simulink model "Ladder_Model"  (R2021b)
settings: Solver=VariableStepAuto  StartTime=0.0  StopTime=0.00005  RelTol=1e-3
model workspace (MAT data in the model file):
  f = [1 10010011.009 20020021.018 30030031.027 40040041.036 50050051.045 60060061.0541 70070071.0631 80080081.0721 90090091.0811 100100101.09 110110111.099 ... (1000 elements, 1x1000)]
  f1 = 120
  fff = Simulink.Parameter
  fff.DataType = 'auto'
  fff.Min = 0
  fff.Max = 100000
  fff.Complexity = 'real'
  fff.Dimensions = [0 0]
undefined symbols (not defined in the file or in its folder): c0, ct0, ct1, ct2, ct3, ct4, cu, cv, frequence
libraries: spsSeriesRLCBranchLib x190, spsGroundLib x49, spsControlledVoltageSourceLib x6, spsImpedanceMeasurementLib x6, spspowerguiLib x1
(part 1 of 2)
settings Model: Creator=anyon  LastModifiedBy=anyon
settings DebuggingCC: UnconnectedInputMsg=none  UnconnectedOutputMsg=none  UnconnectedLineMsg=none

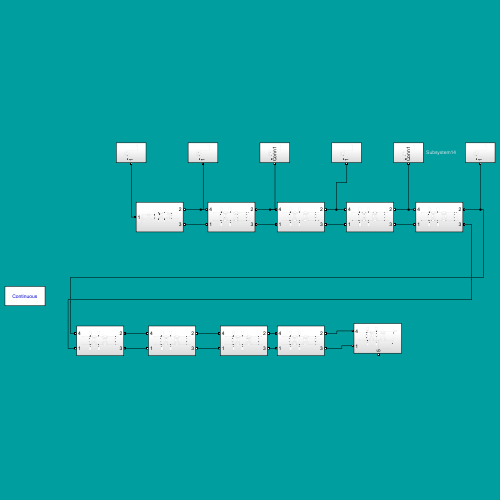
[thumbnail: Simulink's stored preview of the top-level diagram]
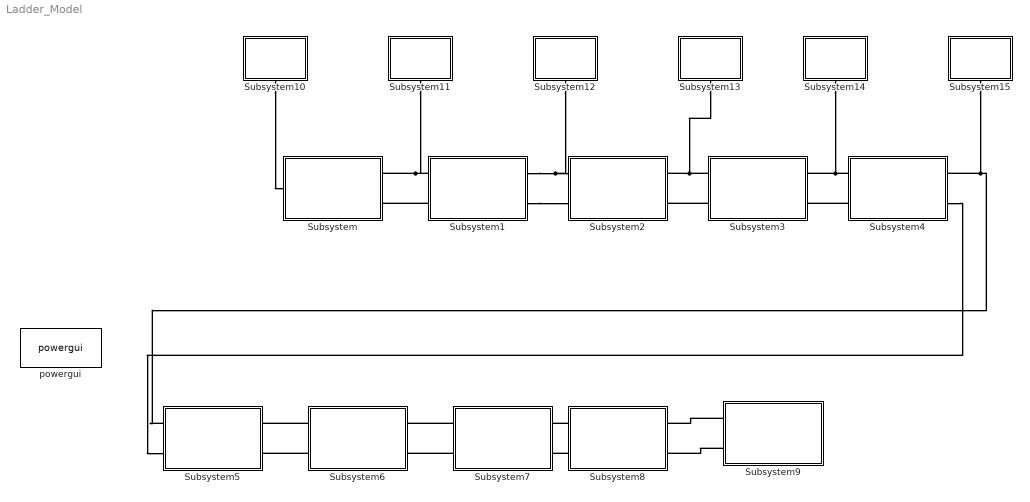
== system Ladder_Model ==
  Subsystem : Subsystem
  Subsystem1 : Subsystem
  Subsystem10 : Subsystem
  Subsystem11 : Subsystem
  Subsystem12 : Subsystem
  Subsystem13 : Subsystem
  Subsystem14 : Subsystem
  Subsystem15 : Subsystem
  Subsystem2 : Subsystem
  Subsystem3 : Subsystem
  Subsystem4 : Subsystem
  Subsystem5 : Subsystem
  Subsystem6 : Subsystem
  Subsystem7 : Subsystem
  Subsystem8 : Subsystem
  Subsystem9 : Subsystem
      settings: PortSchema="{\"entries\":[{\"content\":{\"sides\":[{\"content\":{\"connectorIds\":[\"LConn1\",\"LConn2\"]},\"type\":\"ConnectorPlacement.EquallySpacedRectSide\",\"uuid\":\"888d1c52-7aed-44f6-9b96-844e68c0057c\"},{\"content\":{\"connectorIds\":[],\"side\":\"RIGHT\"},\"type\":\"ConnectorPlacement.EquallySpacedRectSide\",\"uuid\":\"cf946314-0450-4f6f-9852-9e8c811de33d\"},{\"content\":{\"connectorIds\":[],\"side\":\"TOP\"},\"type\":\"ConnectorPlacement.EquallySpacedRectSide\",\"uuid\":\"8536e835-0fb7-4cc6-8052-3a4e7f150ace\"},{\"content\":{\"connectorIds\":[\"RConn1\"],\"side\":\"BOTTOM\"},\"type\":\"ConnectorPlacement.EquallySpacedRectSide\",\"uuid\":\"e79273be-3b6f-4907-8bf0-c99885256dac\"}]},\"type\":\"ConnectorPlacement.EquallySpacedConnector\",\"uuid\":\"3af04479-6e45-456c-916e-cd1a3b349c97\"}],\"packageUris\":[\"http://schema.mathworks.com/mf0/Connector/R2020b\"],\"version\":\"1.0\"}"
  powergui : spspowerguiLib/powergui  Priority=1  SimulationMode=Continuous  SampleTime=50e-6  frequency=60  Iterations=50  frequencyindice=60  Pbase=100e6  ErrMax=1e-4  UnitsV=kV  UnitsW=MW  buscounter=0  FunctionMessages=off  echomessages=off  EnableUseOfTLC=off  CurrentSourceSwitches=off  DisableSnubberDevices=off  DisableRonSwitches=off  DisableVfSwitches=off  DisplayEquations=off  AutomaticDiscreteSolvers=off  SolverType=Tustin/Backward Euler (TBE)  Interpol=off  ExternalGateDelay=off  methode=off  Ts=100  x0status=blocks  SPID=on  SwTol=0  HookPort=off  NonlinearTolerance=1e-4  nMaxIteration=100  ContinueOnMaxIteration=off  RestoreLinks=warning  ResistiveCurrentMeasurement=off  Frange=[0:2:500]  Ylog=off  Xlog=on  ShowGrid=off  save=off  variable=ZData  structure=0  ZoomFFT=off  StartTime=0.0  cycles=1  DisplayStyle=1  fundamental=60  FreqAxis=off  MaxFrequency=1000  frequencyindicesteady=1  RmsSteady=1  display=off
  connections:
  Subsystem1/RConn1 -- Subsystem12/LConn1 -- Subsystem2/LConn1
  Subsystem1/RConn2 -- Subsystem2/LConn2
  Subsystem3/LConn2 -- Subsystem2/RConn2
  Subsystem3/LConn1 -- Subsystem13/LConn1 -- Subsystem2/RConn1
  Subsystem1/LConn2 -- Subsystem/RConn2
  Subsystem1/LConn1 -- Subsystem/RConn1 -- Subsystem11/LConn1
  Subsystem7/LConn1 -- Subsystem6/RConn1
  Subsystem4/RConn2 -- Subsystem5/LConn2
  Subsystem6/LConn1 -- Subsystem5/RConn1
  Subsystem6/LConn2 -- Subsystem5/RConn2
  Subsystem7/LConn2 -- Subsystem6/RConn2
  Subsystem5/LConn1 -- Subsystem15/LConn1 -- Subsystem4/RConn1
  Subsystem4/LConn1 -- Subsystem14/LConn1 -- Subsystem3/RConn1
  Subsystem4/LConn2 -- Subsystem3/RConn2
  Subsystem9/LConn1 -- Subsystem8/RConn1
  Subsystem9/LConn2 -- Subsystem8/RConn2
  Subsystem8/LConn2 -- Subsystem7/RConn2
  Subsystem8/LConn1 -- Subsystem7/RConn1
  Subsystem10/LConn1 -- Subsystem/LConn1

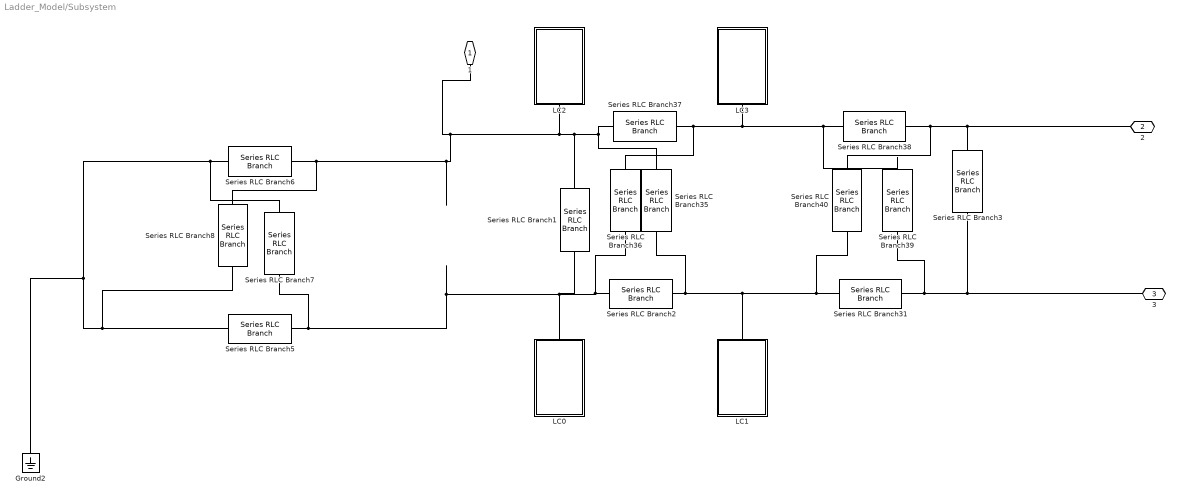
== system Ladder_Model/Subsystem ==
  Ground2 : spsGroundLib/Ground  LConnTagsString=a
  LC0 : Subsystem
  LC1 : Subsystem
  LC2 : Subsystem
  LC3 : Subsystem
  Series RLC Branch1 : spsSeriesRLCBranchLib/Series RLC Branch  LConnTagsString=__new0  RConnTagsString=__new0  BranchType=C  Resistance=1  Inductance=1e-6  SetiL0=off  InitialCurrent=0  Capacitance=ct0  Setx0=off  InitialVoltage=0  Measurements=Branch voltage and current
  Series RLC Branch2 : spsSeriesRLCBranchLib/Series RLC Branch  LConnTagsString=__new0  RConnTagsString=__new0  BranchType=C  Resistance=1  Inductance=1e-6  SetiL0=off  InitialCurrent=0  Capacitance=cu  Setx0=off  InitialVoltage=0  Measurements=None
  Series RLC Branch3 : spsSeriesRLCBranchLib/Series RLC Branch  LConnTagsString=__new0  RConnTagsString=__new0  BranchType=C  Resistance=1  Inductance=1e-6  SetiL0=off  InitialCurrent=0  Capacitance=ct0  Setx0=off  InitialVoltage=0  Measurements=None
  Series RLC Branch{5..6,31,38} (4 alike) : spsSeriesRLCBranchLib/Series RLC Branch  LConnTagsString=__new0  RConnTagsString=__new0  BranchType=C  Resistance=1  Inductance=1e-6  SetiL0=off  InitialCurrent=0  Capacitance=cv  Setx0=off  InitialVoltage=0  Measurements=None
  Series RLC Branch35 : spsSeriesRLCBranchLib/Series RLC Branch  LConnTagsString=__new0  RConnTagsString=__new0  BranchType=C  Resistance=1  Inductance=1e-6  SetiL0=off  InitialCurrent=0  Capacitance=ct2  Setx0=off  InitialVoltage=0  Measurements=None
  Series RLC Branch36 : spsSeriesRLCBranchLib/Series RLC Branch  LConnTagsString=__new0  RConnTagsString=__new0  BranchType=C  Resistance=1  Inductance=1e-6  SetiL0=off  InitialCurrent=0  Capacitance=ct1  Setx0=off  InitialVoltage=0  Measurements=None
  Series RLC Branch37 : spsSeriesRLCBranchLib/Series RLC Branch  LConnTagsString=__new0  RConnTagsString=__new0  BranchType=C  Resistance=1  Inductance=1e-6  SetiL0=off  InitialCurrent=0  Capacitance=cu  Setx0=off  InitialVoltage=0  Measurements=None
  Series RLC Branch39 : spsSeriesRLCBranchLib/Series RLC Branch  LConnTagsString=__new0  RConnTagsString=__new0  BranchType=C  Resistance=1  Inductance=1e-6  SetiL0=off  InitialCurrent=0  Capacitance=ct4  Setx0=off  InitialVoltage=0  Measurements=None
  Series RLC Branch40 : spsSeriesRLCBranchLib/Series RLC Branch  LConnTagsString=__new0  RConnTagsString=__new0  BranchType=C  Resistance=1  Inductance=1e-6  SetiL0=off  InitialCurrent=0  Capacitance=ct3  Setx0=off  InitialVoltage=0  Measurements=None
  Series RLC Branch7 : spsSeriesRLCBranchLib/Series RLC Branch  LConnTagsString=__new0  RConnTagsString=__new0  BranchType=C  Resistance=1  Inductance=1e-6  SetiL0=off  InitialCurrent=0  Capacitance=ct4  Setx0=off  InitialVoltage=0  Measurements=None
  Series RLC Branch8 : spsSeriesRLCBranchLib/Series RLC Branch  LConnTagsString=__new0  RConnTagsString=__new0  BranchType=C  Resistance=1  Inductance=1e-6  SetiL0=off  InitialCurrent=0  Capacitance=ct3  Setx0=off  InitialVoltage=0  Measurements=None
  1 : PMIOPort  Side=Left
  2 : PMIOPort  Port=2  Side=Right
  3 : PMIOPort  Port=3  Side=Right
  connections:
  Series RLC Branch31/RConn1 -- Series RLC Branch39/RConn1 -- 3/RConn1 -- Series RLC Branch3/LConn1
  Series RLC Branch37/RConn1 -- Series RLC Branch36/RConn1 -- Series RLC Branch39/LConn1 -- Series RLC Branch38/LConn1 -- LC3/LConn1
  Series RLC Branch6/RConn1 -- Series RLC Branch1/RConn1 -- Series RLC Branch37/LConn1 -- Series RLC Branch35/LConn1 -- LC2/LConn1 -- 1/RConn1 -- Series RLC Branch8/RConn1
  Series RLC Branch2/RConn1 -- Series RLC Branch35/RConn1 -- Series RLC Branch40/LConn1 -- Series RLC Branch31/LConn1 -- LC1/LConn1
  Series RLC Branch38/RConn1 -- 2/RConn1 -- Series RLC Branch3/RConn1 -- Series RLC Branch40/RConn1
  Series RLC Branch2/LConn1 -- Series RLC Branch7/RConn1 -- Series RLC Branch5/RConn1 -- Series RLC Branch1/LConn1 -- LC0/LConn1 -- Series RLC Branch36/LConn1
  Series RLC Branch5/LConn1 -- Ground2/LConn1 -- Series RLC Branch7/LConn1 -- Series RLC Branch6/LConn1 -- Series RLC Branch8/LConn1

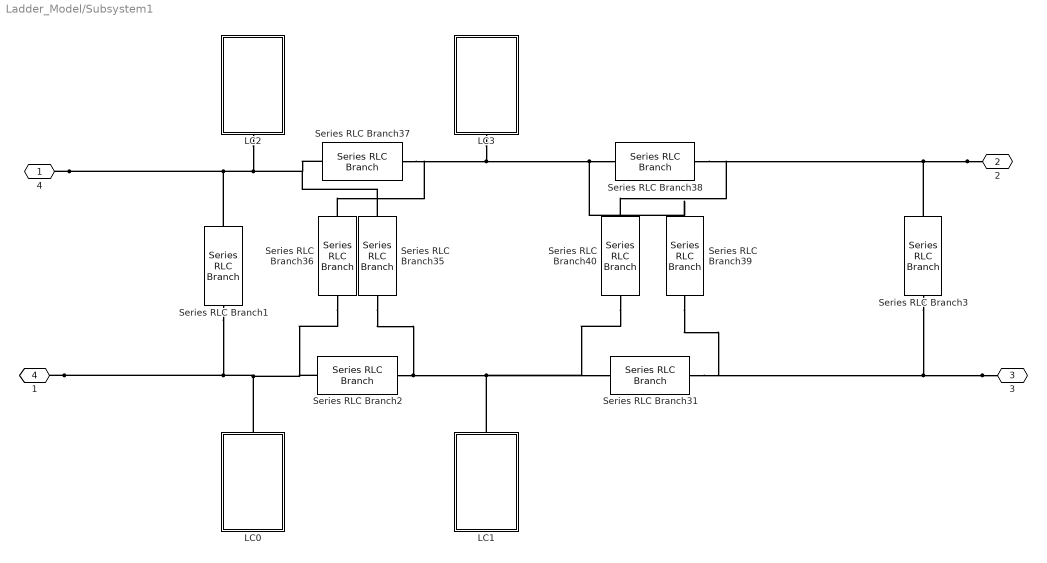
== system Ladder_Model/Subsystem1 ==
  LC0 : Subsystem
  LC1 : Subsystem
  LC2 : Subsystem
  LC3 : Subsystem
  Series RLC Branch1 : spsSeriesRLCBranchLib/Series RLC Branch  LConnTagsString=__new0  RConnTagsString=__new0  BranchType=C  Resistance=1  Inductance=1e-6  SetiL0=off  InitialCurrent=0  Capacitance=ct0  Setx0=off  InitialVoltage=0  Measurements=None
  Series RLC Branch2 : spsSeriesRLCBranchLib/Series RLC Branch  LConnTagsString=__new0  RConnTagsString=__new0  BranchType=C  Resistance=1  Inductance=1e-6  SetiL0=off  InitialCurrent=0  Capacitance=cu  Setx0=off  InitialVoltage=0  Measurements=None
  Series RLC Branch3 : spsSeriesRLCBranchLib/Series RLC Branch  LConnTagsString=__new0  RConnTagsString=__new0  BranchType=C  Resistance=1  Inductance=1e-6  SetiL0=off  InitialCurrent=0  Capacitance=ct0  Setx0=off  InitialVoltage=0  Measurements=None
  Series RLC Branch31 : spsSeriesRLCBranchLib/Series RLC Branch  LConnTagsString=__new0  RConnTagsString=__new0  BranchType=C  Resistance=1  Inductance=1e-6  SetiL0=off  InitialCurrent=0  Capacitance=cv  Setx0=off  InitialVoltage=0  Measurements=None
  Series RLC Branch35 : spsSeriesRLCBranchLib/Series RLC Branch  LConnTagsString=__new0  RConnTagsString=__new0  BranchType=C  Resistance=1  Inductance=1e-6  SetiL0=off  InitialCurrent=0  Capacitance=ct2  Setx0=off  InitialVoltage=0  Measurements=None
  Series RLC Branch36 : spsSeriesRLCBranchLib/Series RLC Branch  LConnTagsString=__new0  RConnTagsString=__new0  BranchType=C  Resistance=1  Inductance=1e-6  SetiL0=off  InitialCurrent=0  Capacitance=ct1  Setx0=off  InitialVoltage=0  Measurements=None
  Series RLC Branch37 : spsSeriesRLCBranchLib/Series RLC Branch  LConnTagsString=__new0  RConnTagsString=__new0  BranchType=C  Resistance=1  Inductance=1e-6  SetiL0=off  InitialCurrent=0  Capacitance=cu  Setx0=off  InitialVoltage=0  Measurements=None
  Series RLC Branch38 : spsSeriesRLCBranchLib/Series RLC Branch  LConnTagsString=__new0  RConnTagsString=__new0  BranchType=C  Resistance=1  Inductance=1e-6  SetiL0=off  InitialCurrent=0  Capacitance=cv  Setx0=off  InitialVoltage=0  Measurements=None
  Series RLC Branch39 : spsSeriesRLCBranchLib/Series RLC Branch  LConnTagsString=__new0  RConnTagsString=__new0  BranchType=C  Resistance=1  Inductance=1e-6  SetiL0=off  InitialCurrent=0  Capacitance=ct4  Setx0=off  InitialVoltage=0  Measurements=None
  Series RLC Branch40 : spsSeriesRLCBranchLib/Series RLC Branch  LConnTagsString=__new0  RConnTagsString=__new0  BranchType=C  Resistance=1  Inductance=1e-6  SetiL0=off  InitialCurrent=0  Capacitance=ct3  Setx0=off  InitialVoltage=0  Measurements=None
  4 : PMIOPort  Side=Left
  2 : PMIOPort  Port=2  Side=Right
  3 : PMIOPort  Port=3  Side=Right
  1 : PMIOPort  Port=4  Side=Left
  connections:
  3/RConn1 -- Series RLC Branch39/RConn1 -- Series RLC Branch31/RConn1 -- Series RLC Branch3/LConn1
  Series RLC Branch39/LConn1 -- Series RLC Branch38/LConn1 -- Series RLC Branch37/RConn1 -- Series RLC Branch36/RConn1 -- LC3/LConn1
  4/RConn1 -- Series RLC Branch37/LConn1 -- Series RLC Branch35/LConn1 -- LC2/LConn1 -- Series RLC Branch1/RConn1
  Series RLC Branch35/RConn1 -- Series RLC Branch2/RConn1 -- LC1/LConn1 -- Series RLC Branch40/LConn1 -- Series RLC Branch31/LConn1
  2/RConn1 -- Series RLC Branch40/RConn1 -- Series RLC Branch38/RConn1 -- Series RLC Branch3/RConn1
  1/RConn1 -- Series RLC Branch36/LConn1 -- Series RLC Branch2/LConn1 -- LC0/LConn1 -- Series RLC Branch1/LConn1

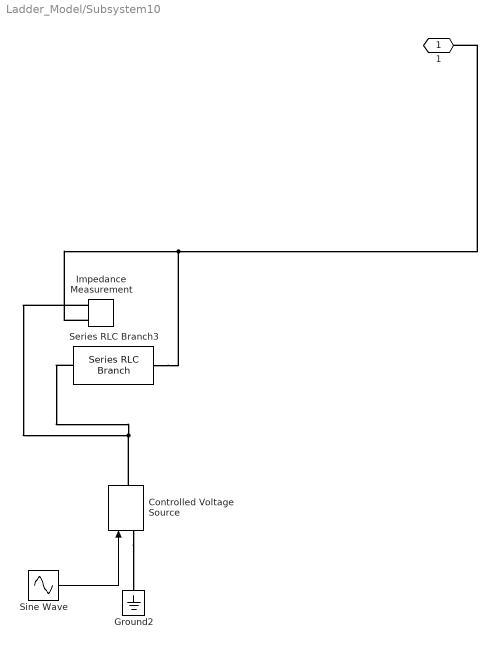
== system Ladder_Model/Subsystem10 ==
  Controlled Voltage Source : spsControlledVoltageSourceLib/Controlled Voltage Source  Initialize=on  Source_Type=AC  Amplitude=120  Phase=0  Frequency=60  Measurements=None
  Ground2 : spsGroundLib/Ground  LConnTagsString=a
  Impedance Measurement : spsImpedanceMeasurementLib/Impedance Measurement  LConnTagsString=+|-  Factor=1
      settings: SourceProductBaseCode=PS
  Series RLC Branch3 : spsSeriesRLCBranchLib/Series RLC Branch  LConnTagsString=__new0  RConnTagsString=__new0  BranchType=R  Resistance=100  Inductance=1e-6  SetiL0=off  InitialCurrent=0  Capacitance=1e-6  Setx0=off  InitialVoltage=0  Measurements=None
  Sine Wave : Sin  Amplitude=frequence  Frequency=0  SampleTime=10
  1 : PMIOPort  Side=Left
  wires:
  Sine Wave/1 -> Controlled Voltage Source/1
  connections:
  Series RLC Branch3/LConn1 -- Impedance Measurement/LConn2 -- 1/RConn1
  Impedance Measurement/LConn1 -- Controlled Voltage Source/RConn1 -- Series RLC Branch3/RConn1
  Controlled Voltage Source/LConn1 -- Ground2/LConn1

== system Ladder_Model/Subsystem11 ==
  Controlled Voltage Source : spsControlledVoltageSourceLib/Controlled Voltage Source  Initialize=on  Source_Type=AC  Amplitude=120  Phase=0  Frequency=60  Measurements=None
  Ground2 : spsGroundLib/Ground  LConnTagsString=a
  Impedance Measurement : spsImpedanceMeasurementLib/Impedance Measurement  LConnTagsString=+|-  Factor=1
      settings: SourceProductBaseCode=PS
  Series RLC Branch3 : spsSeriesRLCBranchLib/Series RLC Branch  LConnTagsString=__new0  RConnTagsString=__new0  BranchType=R  Resistance=100  Inductance=1e-6  SetiL0=off  InitialCurrent=0  Capacitance=1e-6  Setx0=off  InitialVoltage=0  Measurements=None
  Sine Wave : Sin  Amplitude=frequence  Frequency=0  SampleTime=10
  1 : PMIOPort  Side=Left
  wires:
  Sine Wave/1 -> Controlled Voltage Source/1
  connections:
  Impedance Measurement/LConn2 -- Series RLC Branch3/LConn1 -- 1/RConn1
  Series RLC Branch3/RConn1 -- Impedance Measurement/LConn1 -- Controlled Voltage Source/RConn1
  Controlled Voltage Source/LConn1 -- Ground2/LConn1

== system Ladder_Model/Subsystem12 ==
  Controlled Voltage Source : spsControlledVoltageSourceLib/Controlled Voltage Source  Initialize=on  Source_Type=AC  Amplitude=120  Phase=0  Frequency=60  Measurements=None
  Ground2 : spsGroundLib/Ground  LConnTagsString=a
  Impedance Measurement : spsImpedanceMeasurementLib/Impedance Measurement  LConnTagsString=+|-  Factor=1
      settings: SourceProductBaseCode=PS
  Series RLC Branch3 : spsSeriesRLCBranchLib/Series RLC Branch  LConnTagsString=__new0  RConnTagsString=__new0  BranchType=R  Resistance=100  Inductance=1e-6  SetiL0=off  InitialCurrent=0  Capacitance=1e-6  Setx0=off  InitialVoltage=0  Measurements=None
  Sine Wave : Sin  Amplitude=frequence  Frequency=0  SampleTime=10
  Conn1 : PMIOPort  Side=Left
  wires:
  Sine Wave/1 -> Controlled Voltage Source/1
  connections:
  Impedance Measurement/LConn2 -- Series RLC Branch3/LConn1 -- Conn1/RConn1
  Series RLC Branch3/RConn1 -- Impedance Measurement/LConn1 -- Controlled Voltage Source/RConn1
  Controlled Voltage Source/LConn1 -- Ground2/LConn1

== system Ladder_Model/Subsystem13 ==
  Controlled Voltage Source : spsControlledVoltageSourceLib/Controlled Voltage Source  Initialize=on  Source_Type=AC  Amplitude=120  Phase=0  Frequency=60  Measurements=None
  Ground2 : spsGroundLib/Ground  LConnTagsString=a
  Impedance Measurement : spsImpedanceMeasurementLib/Impedance Measurement  LConnTagsString=+|-  Factor=1
      settings: SourceProductBaseCode=PS
  Series RLC Branch3 : spsSeriesRLCBranchLib/Series RLC Branch  LConnTagsString=__new0  RConnTagsString=__new0  BranchType=R  Resistance=100  Inductance=1e-6  SetiL0=off  InitialCurrent=0  Capacitance=1e-6  Setx0=off  InitialVoltage=0  Measurements=None
  Sine Wave : Sin  Amplitude=frequence  Frequency=0  SampleTime=10
  1 : PMIOPort  Side=Left
  wires:
  Sine Wave/1 -> Controlled Voltage Source/1
  connections:
  Impedance Measurement/LConn2 -- Series RLC Branch3/LConn1 -- 1/RConn1
  Series RLC Branch3/RConn1 -- Impedance Measurement/LConn1 -- Controlled Voltage Source/RConn1
  Controlled Voltage Source/LConn1 -- Ground2/LConn1

== system Ladder_Model/Subsystem14 ==
  Controlled Voltage Source : spsControlledVoltageSourceLib/Controlled Voltage Source  Initialize=on  Source_Type=AC  Amplitude=120  Phase=0  Frequency=60  Measurements=None
  Ground2 : spsGroundLib/Ground  LConnTagsString=a
  Impedance Measurement : spsImpedanceMeasurementLib/Impedance Measurement  LConnTagsString=+|-  Factor=1
      settings: SourceProductBaseCode=PS
  Series RLC Branch3 : spsSeriesRLCBranchLib/Series RLC Branch  LConnTagsString=__new0  RConnTagsString=__new0  BranchType=R  Resistance=100  Inductance=1e-6  SetiL0=off  InitialCurrent=0  Capacitance=1e-6  Setx0=off  InitialVoltage=0  Measurements=None
  Sine Wave : Sin  Amplitude=frequence  Frequency=0  SampleTime=10
  Conn1 : PMIOPort  Side=Left
  wires:
  Sine Wave/1 -> Controlled Voltage Source/1
  connections:
  Impedance Measurement/LConn2 -- Series RLC Branch3/LConn1 -- Conn1/RConn1
  Series RLC Branch3/RConn1 -- Impedance Measurement/LConn1 -- Controlled Voltage Source/RConn1
  Controlled Voltage Source/LConn1 -- Ground2/LConn1

== system Ladder_Model/Subsystem15 ==
  Controlled Voltage Source : spsControlledVoltageSourceLib/Controlled Voltage Source  Initialize=on  Source_Type=AC  Amplitude=120  Phase=0  Frequency=60  Measurements=None
  Ground2 : spsGroundLib/Ground  LConnTagsString=a
  Impedance Measurement : spsImpedanceMeasurementLib/Impedance Measurement  LConnTagsString=+|-  Factor=1
      settings: SourceProductBaseCode=PS
  Series RLC Branch3 : spsSeriesRLCBranchLib/Series RLC Branch  LConnTagsString=__new0  RConnTagsString=__new0  BranchType=R  Resistance=100  Inductance=1e-6  SetiL0=off  InitialCurrent=0  Capacitance=1e-6  Setx0=off  InitialVoltage=0  Measurements=None
  Sine Wave : Sin  Amplitude=frequence  Frequency=0  SampleTime=10
  1 : PMIOPort  Side=Left
  wires:
  Sine Wave/1 -> Controlled Voltage Source/1
  connections:
  Impedance Measurement/LConn2 -- Series RLC Branch3/LConn1 -- 1/RConn1
  Series RLC Branch3/RConn1 -- Impedance Measurement/LConn1 -- Controlled Voltage Source/RConn1
  Controlled Voltage Source/LConn1 -- Ground2/LConn1

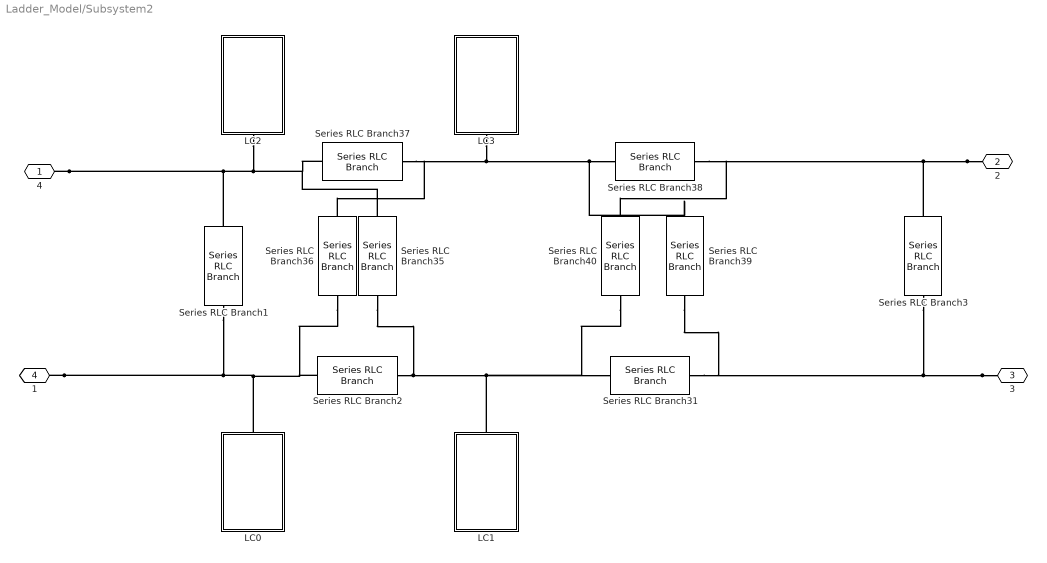
== system Ladder_Model/Subsystem2 ==
  LC0 : Subsystem
  LC1 : Subsystem
  LC2 : Subsystem
  LC3 : Subsystem
  Series RLC Branch1 : spsSeriesRLCBranchLib/Series RLC Branch  LConnTagsString=__new0  RConnTagsString=__new0  BranchType=C  Resistance=1  Inductance=1e-6  SetiL0=off  InitialCurrent=0  Capacitance=ct0  Setx0=off  InitialVoltage=0  Measurements=None
  Series RLC Branch2 : spsSeriesRLCBranchLib/Series RLC Branch  LConnTagsString=__new0  RConnTagsString=__new0  BranchType=C  Resistance=1  Inductance=1e-6  SetiL0=off  InitialCurrent=0  Capacitance=cu  Setx0=off  InitialVoltage=0  Measurements=None
  Series RLC Branch3 : spsSeriesRLCBranchLib/Series RLC Branch  LConnTagsString=__new0  RConnTagsString=__new0  BranchType=C  Resistance=1  Inductance=1e-6  SetiL0=off  InitialCurrent=0  Capacitance=ct0  Setx0=off  InitialVoltage=0  Measurements=None
  Series RLC Branch31 : spsSeriesRLCBranchLib/Series RLC Branch  LConnTagsString=__new0  RConnTagsString=__new0  BranchType=C  Resistance=1  Inductance=1e-6  SetiL0=off  InitialCurrent=0  Capacitance=cv  Setx0=off  InitialVoltage=0  Measurements=None
  Series RLC Branch35 : spsSeriesRLCBranchLib/Series RLC Branch  LConnTagsString=__new0  RConnTagsString=__new0  BranchType=C  Resistance=1  Inductance=1e-6  SetiL0=off  InitialCurrent=0  Capacitance=ct2  Setx0=off  InitialVoltage=0  Measurements=None
  Series RLC Branch36 : spsSeriesRLCBranchLib/Series RLC Branch  LConnTagsString=__new0  RConnTagsString=__new0  BranchType=C  Resistance=1  Inductance=1e-6  SetiL0=off  InitialCurrent=0  Capacitance=ct1  Setx0=off  InitialVoltage=0  Measurements=None
  Series RLC Branch37 : spsSeriesRLCBranchLib/Series RLC Branch  LConnTagsString=__new0  RConnTagsString=__new0  BranchType=C  Resistance=1  Inductance=1e-6  SetiL0=off  InitialCurrent=0  Capacitance=cu  Setx0=off  InitialVoltage=0  Measurements=None
  Series RLC Branch38 : spsSeriesRLCBranchLib/Series RLC Branch  LConnTagsString=__new0  RConnTagsString=__new0  BranchType=C  Resistance=1  Inductance=1e-6  SetiL0=off  InitialCurrent=0  Capacitance=cv  Setx0=off  InitialVoltage=0  Measurements=None
  Series RLC Branch39 : spsSeriesRLCBranchLib/Series RLC Branch  LConnTagsString=__new0  RConnTagsString=__new0  BranchType=C  Resistance=1  Inductance=1e-6  SetiL0=off  InitialCurrent=0  Capacitance=ct4  Setx0=off  InitialVoltage=0  Measurements=None
  Series RLC Branch40 : spsSeriesRLCBranchLib/Series RLC Branch  LConnTagsString=__new0  RConnTagsString=__new0  BranchType=C  Resistance=1  Inductance=1e-6  SetiL0=off  InitialCurrent=0  Capacitance=ct3  Setx0=off  InitialVoltage=0  Measurements=None
  4 : PMIOPort  Side=Left
  2 : PMIOPort  Port=2  Side=Right
  3 : PMIOPort  Port=3  Side=Right
  1 : PMIOPort  Port=4  Side=Left
  connections:
  3/RConn1 -- Series RLC Branch39/RConn1 -- Series RLC Branch31/RConn1 -- Series RLC Branch3/LConn1
  Series RLC Branch39/LConn1 -- Series RLC Branch38/LConn1 -- Series RLC Branch37/RConn1 -- Series RLC Branch36/RConn1 -- LC3/LConn1
  4/RConn1 -- Series RLC Branch37/LConn1 -- Series RLC Branch35/LConn1 -- LC2/LConn1 -- Series RLC Branch1/RConn1
  Series RLC Branch35/RConn1 -- Series RLC Branch2/RConn1 -- LC1/LConn1 -- Series RLC Branch40/LConn1 -- Series RLC Branch31/LConn1
  2/RConn1 -- Series RLC Branch40/RConn1 -- Series RLC Branch38/RConn1 -- Series RLC Branch3/RConn1
  1/RConn1 -- Series RLC Branch36/LConn1 -- Series RLC Branch2/LConn1 -- LC0/LConn1 -- Series RLC Branch1/LConn1

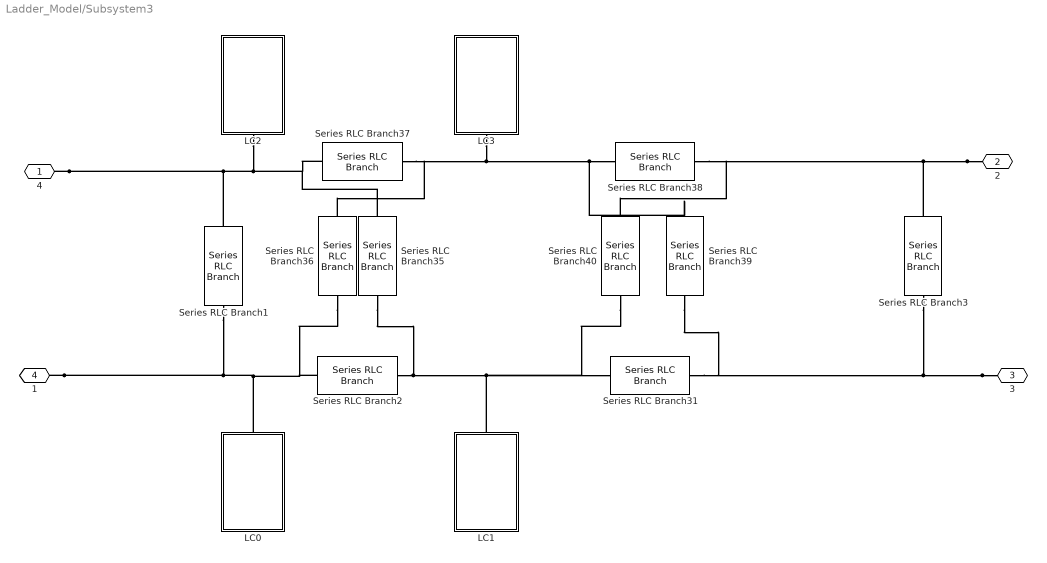
== system Ladder_Model/Subsystem3 ==
  LC0 : Subsystem
  LC1 : Subsystem
  LC2 : Subsystem
  LC3 : Subsystem
  Series RLC Branch1 : spsSeriesRLCBranchLib/Series RLC Branch  LConnTagsString=__new0  RConnTagsString=__new0  BranchType=C  Resistance=1  Inductance=1e-6  SetiL0=off  InitialCurrent=0  Capacitance=ct0  Setx0=off  InitialVoltage=0  Measurements=None
  Series RLC Branch2 : spsSeriesRLCBranchLib/Series RLC Branch  LConnTagsString=__new0  RConnTagsString=__new0  BranchType=C  Resistance=1  Inductance=1e-6  SetiL0=off  InitialCurrent=0  Capacitance=cu  Setx0=off  InitialVoltage=0  Measurements=None
  Series RLC Branch3 : spsSeriesRLCBranchLib/Series RLC Branch  LConnTagsString=__new0  RConnTagsString=__new0  BranchType=C  Resistance=1  Inductance=1e-6  SetiL0=off  InitialCurrent=0  Capacitance=ct0  Setx0=off  InitialVoltage=0  Measurements=None
  Series RLC Branch31 : spsSeriesRLCBranchLib/Series RLC Branch  LConnTagsString=__new0  RConnTagsString=__new0  BranchType=C  Resistance=1  Inductance=1e-6  SetiL0=off  InitialCurrent=0  Capacitance=cv  Setx0=off  InitialVoltage=0  Measurements=None
  Series RLC Branch35 : spsSeriesRLCBranchLib/Series RLC Branch  LConnTagsString=__new0  RConnTagsString=__new0  BranchType=C  Resistance=1  Inductance=1e-6  SetiL0=off  InitialCurrent=0  Capacitance=ct2  Setx0=off  InitialVoltage=0  Measurements=None
  Series RLC Branch36 : spsSeriesRLCBranchLib/Series RLC Branch  LConnTagsString=__new0  RConnTagsString=__new0  BranchType=C  Resistance=1  Inductance=1e-6  SetiL0=off  InitialCurrent=0  Capacitance=ct1  Setx0=off  InitialVoltage=0  Measurements=None
  Series RLC Branch37 : spsSeriesRLCBranchLib/Series RLC Branch  LConnTagsString=__new0  RConnTagsString=__new0  BranchType=C  Resistance=1  Inductance=1e-6  SetiL0=off  InitialCurrent=0  Capacitance=cu  Setx0=off  InitialVoltage=0  Measurements=None
  Series RLC Branch38 : spsSeriesRLCBranchLib/Series RLC Branch  LConnTagsString=__new0  RConnTagsString=__new0  BranchType=C  Resistance=1  Inductance=1e-6  SetiL0=off  InitialCurrent=0  Capacitance=cv  Setx0=off  InitialVoltage=0  Measurements=None
  Series RLC Branch39 : spsSeriesRLCBranchLib/Series RLC Branch  LConnTagsString=__new0  RConnTagsString=__new0  BranchType=C  Resistance=1  Inductance=1e-6  SetiL0=off  InitialCurrent=0  Capacitance=ct4  Setx0=off  InitialVoltage=0  Measurements=None
  Series RLC Branch40 : spsSeriesRLCBranchLib/Series RLC Branch  LConnTagsString=__new0  RConnTagsString=__new0  BranchType=C  Resistance=1  Inductance=1e-6  SetiL0=off  InitialCurrent=0  Capacitance=ct3  Setx0=off  InitialVoltage=0  Measurements=None
  4 : PMIOPort  Side=Left
  2 : PMIOPort  Port=2  Side=Right
  3 : PMIOPort  Port=3  Side=Right
  1 : PMIOPort  Port=4  Side=Left
  connections:
  3/RConn1 -- Series RLC Branch39/RConn1 -- Series RLC Branch31/RConn1 -- Series RLC Branch3/LConn1
  Series RLC Branch39/LConn1 -- Series RLC Branch38/LConn1 -- Series RLC Branch37/RConn1 -- Series RLC Branch36/RConn1 -- LC3/LConn1
  4/RConn1 -- Series RLC Branch37/LConn1 -- Series RLC Branch35/LConn1 -- LC2/LConn1 -- Series RLC Branch1/RConn1
  Series RLC Branch35/RConn1 -- Series RLC Branch2/RConn1 -- LC1/LConn1 -- Series RLC Branch40/LConn1 -- Series RLC Branch31/LConn1
  2/RConn1 -- Series RLC Branch40/RConn1 -- Series RLC Branch38/RConn1 -- Series RLC Branch3/RConn1
  1/RConn1 -- Series RLC Branch36/LConn1 -- Series RLC Branch2/LConn1 -- LC0/LConn1 -- Series RLC Branch1/LConn1

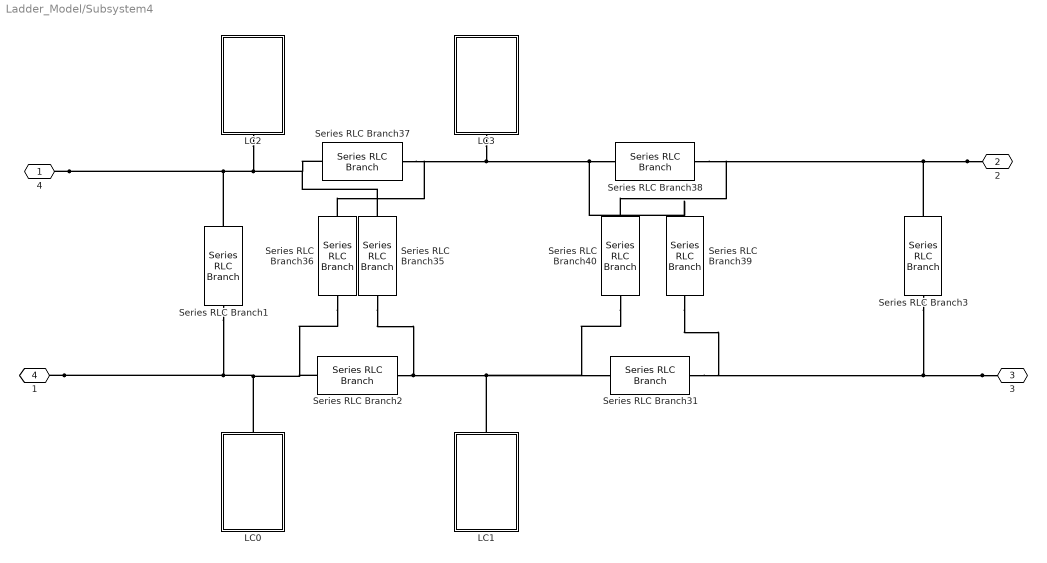
== system Ladder_Model/Subsystem4 ==
  LC0 : Subsystem
  LC1 : Subsystem
  LC2 : Subsystem
  LC3 : Subsystem
  Series RLC Branch1 : spsSeriesRLCBranchLib/Series RLC Branch  LConnTagsString=__new0  RConnTagsString=__new0  BranchType=C  Resistance=1  Inductance=1e-6  SetiL0=off  InitialCurrent=0  Capacitance=ct0  Setx0=off  InitialVoltage=0  Measurements=None
  Series RLC Branch2 : spsSeriesRLCBranchLib/Series RLC Branch  LConnTagsString=__new0  RConnTagsString=__new0  BranchType=C  Resistance=1  Inductance=1e-6  SetiL0=off  InitialCurrent=0  Capacitance=cu  Setx0=off  InitialVoltage=0  Measurements=None
  Series RLC Branch3 : spsSeriesRLCBranchLib/Series RLC Branch  LConnTagsString=__new0  RConnTagsString=__new0  BranchType=C  Resistance=1  Inductance=1e-6  SetiL0=off  InitialCurrent=0  Capacitance=ct0  Setx0=off  InitialVoltage=0  Measurements=None
  Series RLC Branch31 : spsSeriesRLCBranchLib/Series RLC Branch  LConnTagsString=__new0  RConnTagsString=__new0  BranchType=C  Resistance=1  Inductance=1e-6  SetiL0=off  InitialCurrent=0  Capacitance=cv  Setx0=off  InitialVoltage=0  Measurements=None
  Series RLC Branch35 : spsSeriesRLCBranchLib/Series RLC Branch  LConnTagsString=__new0  RConnTagsString=__new0  BranchType=C  Resistance=1  Inductance=1e-6  SetiL0=off  InitialCurrent=0  Capacitance=ct2  Setx0=off  InitialVoltage=0  Measurements=None
  Series RLC Branch36 : spsSeriesRLCBranchLib/Series RLC Branch  LConnTagsString=__new0  RConnTagsString=__new0  BranchType=C  Resistance=1  Inductance=1e-6  SetiL0=off  InitialCurrent=0  Capacitance=ct1  Setx0=off  InitialVoltage=0  Measurements=None
  Series RLC Branch37 : spsSeriesRLCBranchLib/Series RLC Branch  LConnTagsString=__new0  RConnTagsString=__new0  BranchType=C  Resistance=1  Inductance=1e-6  SetiL0=off  InitialCurrent=0  Capacitance=cu  Setx0=off  InitialVoltage=0  Measurements=None
  Series RLC Branch38 : spsSeriesRLCBranchLib/Series RLC Branch  LConnTagsString=__new0  RConnTagsString=__new0  BranchType=C  Resistance=1  Inductance=1e-6  SetiL0=off  InitialCurrent=0  Capacitance=cv  Setx0=off  InitialVoltage=0  Measurements=None
  Series RLC Branch39 : spsSeriesRLCBranchLib/Series RLC Branch  LConnTagsString=__new0  RConnTagsString=__new0  BranchType=C  Resistance=1  Inductance=1e-6  SetiL0=off  InitialCurrent=0  Capacitance=ct4  Setx0=off  InitialVoltage=0  Measurements=None
  Series RLC Branch40 : spsSeriesRLCBranchLib/Series RLC Branch  LConnTagsString=__new0  RConnTagsString=__new0  BranchType=C  Resistance=1  Inductance=1e-6  SetiL0=off  InitialCurrent=0  Capacitance=ct3  Setx0=off  InitialVoltage=0  Measurements=None
  4 : PMIOPort  Side=Left
  2 : PMIOPort  Port=2  Side=Right
  3 : PMIOPort  Port=3  Side=Right
  1 : PMIOPort  Port=4  Side=Left
  connections:
  3/RConn1 -- Series RLC Branch39/RConn1 -- Series RLC Branch31/RConn1 -- Series RLC Branch3/LConn1
  Series RLC Branch39/LConn1 -- Series RLC Branch38/LConn1 -- Series RLC Branch37/RConn1 -- Series RLC Branch36/RConn1 -- LC3/LConn1
  4/RConn1 -- Series RLC Branch37/LConn1 -- Series RLC Branch35/LConn1 -- LC2/LConn1 -- Series RLC Branch1/RConn1
  Series RLC Branch35/RConn1 -- Series RLC Branch2/RConn1 -- LC1/LConn1 -- Series RLC Branch40/LConn1 -- Series RLC Branch31/LConn1
  2/RConn1 -- Series RLC Branch40/RConn1 -- Series RLC Branch38/RConn1 -- Series RLC Branch3/RConn1
  1/RConn1 -- Series RLC Branch36/LConn1 -- Series RLC Branch2/LConn1 -- LC0/LConn1 -- Series RLC Branch1/LConn1

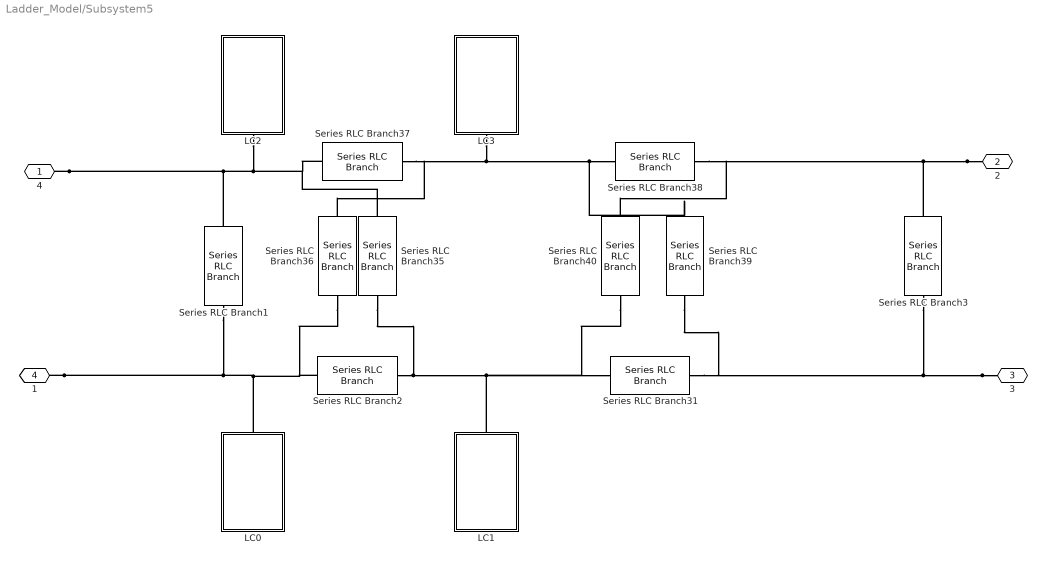
== system Ladder_Model/Subsystem5 ==
  LC0 : Subsystem
  LC1 : Subsystem
  LC2 : Subsystem
  LC3 : Subsystem
  Series RLC Branch1 : spsSeriesRLCBranchLib/Series RLC Branch  LConnTagsString=__new0  RConnTagsString=__new0  BranchType=C  Resistance=1  Inductance=1e-6  SetiL0=off  InitialCurrent=0  Capacitance=ct0  Setx0=off  InitialVoltage=0  Measurements=None
  Series RLC Branch2 : spsSeriesRLCBranchLib/Series RLC Branch  LConnTagsString=__new0  RConnTagsString=__new0  BranchType=C  Resistance=1  Inductance=1e-6  SetiL0=off  InitialCurrent=0  Capacitance=cu  Setx0=off  InitialVoltage=0  Measurements=None
  Series RLC Branch3 : spsSeriesRLCBranchLib/Series RLC Branch  LConnTagsString=__new0  RConnTagsString=__new0  BranchType=C  Resistance=1  Inductance=1e-6  SetiL0=off  InitialCurrent=0  Capacitance=ct0  Setx0=off  InitialVoltage=0  Measurements=None
  Series RLC Branch31 : spsSeriesRLCBranchLib/Series RLC Branch  LConnTagsString=__new0  RConnTagsString=__new0  BranchType=C  Resistance=1  Inductance=1e-6  SetiL0=off  InitialCurrent=0  Capacitance=cv  Setx0=off  InitialVoltage=0  Measurements=None
  Series RLC Branch35 : spsSeriesRLCBranchLib/Series RLC Branch  LConnTagsString=__new0  RConnTagsString=__new0  BranchType=C  Resistance=1  Inductance=1e-6  SetiL0=off  InitialCurrent=0  Capacitance=ct2  Setx0=off  InitialVoltage=0  Measurements=None
  Series RLC Branch36 : spsSeriesRLCBranchLib/Series RLC Branch  LConnTagsString=__new0  RConnTagsString=__new0  BranchType=C  Resistance=1  Inductance=1e-6  SetiL0=off  InitialCurrent=0  Capacitance=ct1  Setx0=off  InitialVoltage=0  Measurements=None
  Series RLC Branch37 : spsSeriesRLCBranchLib/Series RLC Branch  LConnTagsString=__new0  RConnTagsString=__new0  BranchType=C  Resistance=1  Inductance=1e-6  SetiL0=off  InitialCurrent=0  Capacitance=cu  Setx0=off  InitialVoltage=0  Measurements=None
  Series RLC Branch38 : spsSeriesRLCBranchLib/Series RLC Branch  LConnTagsString=__new0  RConnTagsString=__new0  BranchType=C  Resistance=1  Inductance=1e-6  SetiL0=off  InitialCurrent=0  Capacitance=cv  Setx0=off  InitialVoltage=0  Measurements=None
  Series RLC Branch39 : spsSeriesRLCBranchLib/Series RLC Branch  LConnTagsString=__new0  RConnTagsString=__new0  BranchType=C  Resistance=1  Inductance=1e-6  SetiL0=off  InitialCurrent=0  Capacitance=ct4  Setx0=off  InitialVoltage=0  Measurements=None
  Series RLC Branch40 : spsSeriesRLCBranchLib/Series RLC Branch  LConnTagsString=__new0  RConnTagsString=__new0  BranchType=C  Resistance=1  Inductance=1e-6  SetiL0=off  InitialCurrent=0  Capacitance=ct3  Setx0=off  InitialVoltage=0  Measurements=None
  4 : PMIOPort  Side=Left
  2 : PMIOPort  Port=2  Side=Right
  3 : PMIOPort  Port=3  Side=Right
  1 : PMIOPort  Port=4  Side=Left
  connections:
  3/RConn1 -- Series RLC Branch39/RConn1 -- Series RLC Branch31/RConn1 -- Series RLC Branch3/LConn1
  Series RLC Branch39/LConn1 -- Series RLC Branch38/LConn1 -- Series RLC Branch37/RConn1 -- Series RLC Branch36/RConn1 -- LC3/LConn1
  4/RConn1 -- Series RLC Branch37/LConn1 -- Series RLC Branch35/LConn1 -- LC2/LConn1 -- Series RLC Branch1/RConn1
  Series RLC Branch35/RConn1 -- Series RLC Branch2/RConn1 -- LC1/LConn1 -- Series RLC Branch40/LConn1 -- Series RLC Branch31/LConn1
  2/RConn1 -- Series RLC Branch40/RConn1 -- Series RLC Branch38/RConn1 -- Series RLC Branch3/RConn1
  1/RConn1 -- Series RLC Branch36/LConn1 -- Series RLC Branch2/LConn1 -- LC0/LConn1 -- Series RLC Branch1/LConn1

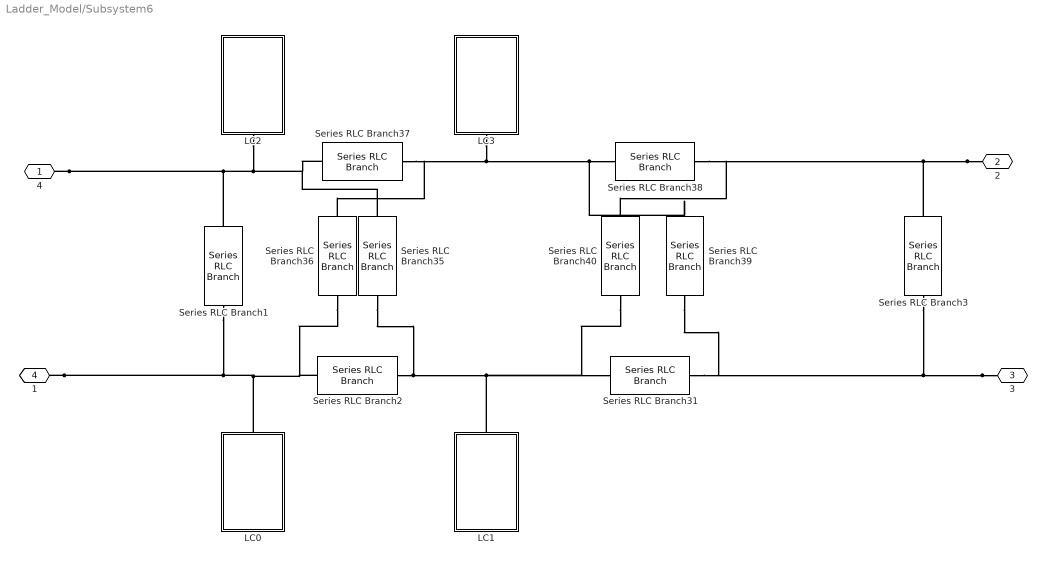
== system Ladder_Model/Subsystem6 ==
  LC0 : Subsystem
  LC1 : Subsystem
  LC2 : Subsystem
  LC3 : Subsystem
  Series RLC Branch1 : spsSeriesRLCBranchLib/Series RLC Branch  LConnTagsString=__new0  RConnTagsString=__new0  BranchType=C  Resistance=1  Inductance=1e-6  SetiL0=off  InitialCurrent=0  Capacitance=ct0  Setx0=off  InitialVoltage=0  Measurements=None
  Series RLC Branch2 : spsSeriesRLCBranchLib/Series RLC Branch  LConnTagsString=__new0  RConnTagsString=__new0  BranchType=C  Resistance=1  Inductance=1e-6  SetiL0=off  InitialCurrent=0  Capacitance=cu  Setx0=off  InitialVoltage=0  Measurements=None
  Series RLC Branch3 : spsSeriesRLCBranchLib/Series RLC Branch  LConnTagsString=__new0  RConnTagsString=__new0  BranchType=C  Resistance=1  Inductance=1e-6  SetiL0=off  InitialCurrent=0  Capacitance=ct0  Setx0=off  InitialVoltage=0  Measurements=None
  Series RLC Branch31 : spsSeriesRLCBranchLib/Series RLC Branch  LConnTagsString=__new0  RConnTagsString=__new0  BranchType=C  Resistance=1  Inductance=1e-6  SetiL0=off  InitialCurrent=0  Capacitance=cv  Setx0=off  InitialVoltage=0  Measurements=None
  Series RLC Branch35 : spsSeriesRLCBranchLib/Series RLC Branch  LConnTagsString=__new0  RConnTagsString=__new0  BranchType=C  Resistance=1  Inductance=1e-6  SetiL0=off  InitialCurrent=0  Capacitance=ct2  Setx0=off  InitialVoltage=0  Measurements=None
  Series RLC Branch36 : spsSeriesRLCBranchLib/Series RLC Branch  LConnTagsString=__new0  RConnTagsString=__new0  BranchType=C  Resistance=1  Inductance=1e-6  SetiL0=off  InitialCurrent=0  Capacitance=ct1  Setx0=off  InitialVoltage=0  Measurements=None
  Series RLC Branch37 : spsSeriesRLCBranchLib/Series RLC Branch  LConnTagsString=__new0  RConnTagsString=__new0  BranchType=C  Resistance=1  Inductance=1e-6  SetiL0=off  InitialCurrent=0  Capacitance=cu  Setx0=off  InitialVoltage=0  Measurements=None
  Series RLC Branch38 : spsSeriesRLCBranchLib/Series RLC Branch  LConnTagsString=__new0  RConnTagsString=__new0  BranchType=C  Resistance=1  Inductance=1e-6  SetiL0=off  InitialCurrent=0  Capacitance=cv  Setx0=off  InitialVoltage=0  Measurements=None
  Series RLC Branch39 : spsSeriesRLCBranchLib/Series RLC Branch  LConnTagsString=__new0  RConnTagsString=__new0  BranchType=C  Resistance=1  Inductance=1e-6  SetiL0=off  InitialCurrent=0  Capacitance=ct4  Setx0=off  InitialVoltage=0  Measurements=None
  Series RLC Branch40 : spsSeriesRLCBranchLib/Series RLC Branch  LConnTagsString=__new0  RConnTagsString=__new0  BranchType=C  Resistance=1  Inductance=1e-6  SetiL0=off  InitialCurrent=0  Capacitance=ct3  Setx0=off  InitialVoltage=0  Measurements=None
  4 : PMIOPort  Side=Left
  2 : PMIOPort  Port=2  Side=Right
  3 : PMIOPort  Port=3  Side=Right
  1 : PMIOPort  Port=4  Side=Left
  connections:
  3/RConn1 -- Series RLC Branch39/RConn1 -- Series RLC Branch31/RConn1 -- Series RLC Branch3/LConn1
  Series RLC Branch39/LConn1 -- Series RLC Branch38/LConn1 -- Series RLC Branch37/RConn1 -- Series RLC Branch36/RConn1 -- LC3/LConn1
  4/RConn1 -- Series RLC Branch37/LConn1 -- Series RLC Branch35/LConn1 -- LC2/LConn1 -- Series RLC Branch1/RConn1
  Series RLC Branch35/RConn1 -- Series RLC Branch2/RConn1 -- LC1/LConn1 -- Series RLC Branch40/LConn1 -- Series RLC Branch31/LConn1
  2/RConn1 -- Series RLC Branch40/RConn1 -- Series RLC Branch38/RConn1 -- Series RLC Branch3/RConn1
  1/RConn1 -- Series RLC Branch36/LConn1 -- Series RLC Branch2/LConn1 -- LC0/LConn1 -- Series RLC Branch1/LConn1
